simulink model "lab3es1ver3"  (R2022a)
settings: Solver=VariableStepAuto  StartTime=0.0  StopTime=10.0  RelTol=1e-3
settings Model: Creator=bonvoltnuovo  LastModifiedBy=bonaventur
settings DebuggingCC: UnconnectedInputMsg=warning  UnconnectedOutputMsg=warning  UnconnectedLineMsg=warning
settings RTWCC: DLArmComputeVersion=19.05

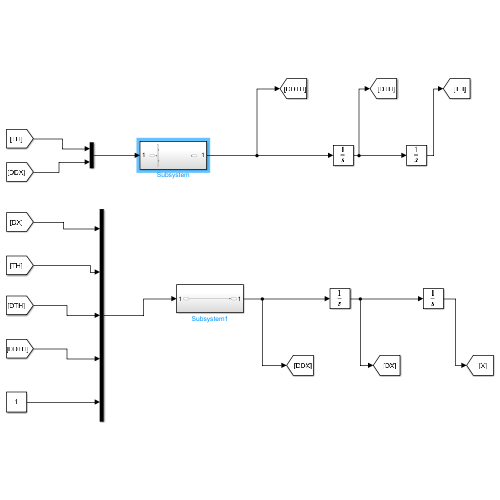
[thumbnail: Simulink's stored preview of the top-level diagram]
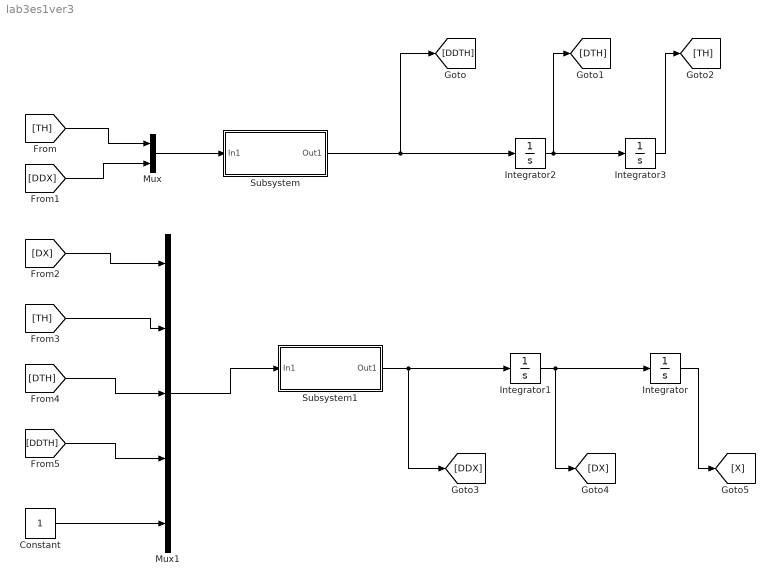
== system lab3es1ver3 ==
  Constant : Constant
  Integrator{,1..3} (4 alike) : Integrator
  Mux : Mux  Inputs=2
  Mux1 : Mux  Inputs=5
  Subsystem : Subsystem
  Subsystem1 : Subsystem
  wires:
  [DDX] -> Mux/2
  Mux/1 -> Subsystem/1(In1)
  [TH] -> Mux/1
  Integrator2/1 -> Integrator3/1, [DTH]
  Integrator3/1 -> [TH]
  Subsystem/1(Out1) -> [DDTH], Integrator2/1
  Constant/1 -> Mux1/5
  [DTH] -> Mux1/3
  [DX] -> Mux1/1
  [DDTH] -> Mux1/4
  Integrator1/1 -> Integrator/1, [DX]
  Integrator/1 -> [X]
  [TH] -> Mux1/2
  Mux1/1 -> Subsystem1/1(In1)
  Subsystem1/1(Out1) -> [DDX], Integrator1/1

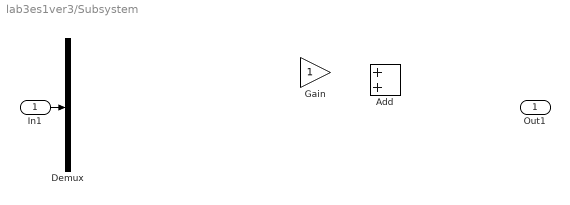
== system lab3es1ver3/Subsystem ==
  In1 : Inport
  Add : Sum
  Demux : Demux  Outputs=2
  Gain : Gain
  Out1 : Outport
  wires:
  In1/1 -> Demux/1

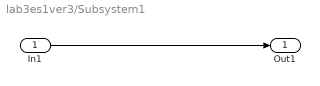
== system lab3es1ver3/Subsystem1 ==
  In1 : Inport
  Out1 : Outport
  wires:
  In1/1 -> Out1/1
